simulink model "FMtest"  (R2025a)
settings: Solver=VariableStepAuto  StartTime=0.0  StopTime=3  RelTol=1e-3
undefined symbols (not defined in the file or in its folder): National_Instruments, PCIe
libraries: sldrtlib x5
settings Model: Creator=simmo536  LastModifiedBy=skaro014
settings DebuggingCC: UnconnectedInputMsg=warning  UnconnectedOutputMsg=warning  UnconnectedLineMsg=warning
settings ModelReferenceCC: EnableRefExpFcnMdlSchedulingChecks=on
settings RTWCC: GPUComputeCapability=3.5  DLArmComputeVersion=19.05

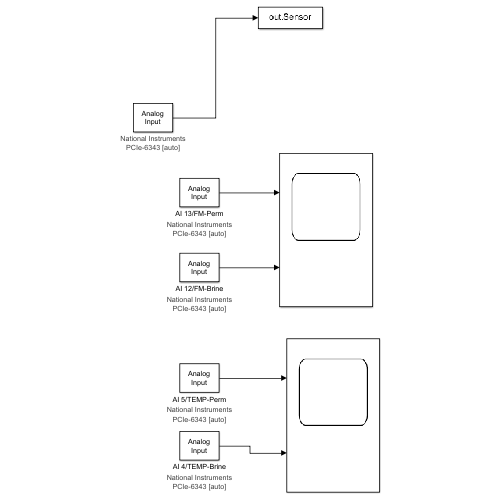
[thumbnail: Simulink's stored preview of the top-level diagram]
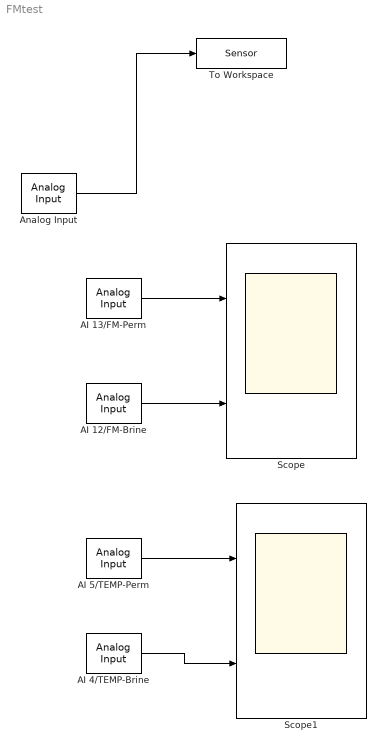
== system FMtest ==
  AI 12/FM-Brine : sldrtlib/Analog Input  SampleTime=0.01  MaxMissedTicks=inf  ShowMissedTicks=off  YieldWhenWaiting=off  DrvName=National_Instruments/PCIe-6343  DrvAddress=4294967295  DrvOptions=[0 0 0 0 0 0 0]  Channels=13  RangeMode=1  VoltRange=1  DataType=2
      settings: AttributesFormatString=National Instruments\nPCIe-6343 [auto]
  AI 13/FM-Perm : sldrtlib/Analog Input  SampleTime=0.01  MaxMissedTicks=inf  ShowMissedTicks=off  YieldWhenWaiting=off  DrvName=National_Instruments/PCIe-6343  DrvAddress=4294967295  DrvOptions=[0 0 0 0 0 0 0]  Channels=14  RangeMode=1  VoltRange=1  DataType=2
      settings: AttributesFormatString=National Instruments\nPCIe-6343 [auto]
  AI 4/TEMP-Brine : sldrtlib/Analog Input  SampleTime=0.01  MaxMissedTicks=inf  ShowMissedTicks=off  YieldWhenWaiting=on  DrvName=National_Instruments/PCIe-6343  DrvAddress=4294967295  DrvOptions=[0 0 0 0 0 0 0]  Channels=5  RangeMode=1  VoltRange=1  DataType=2
      settings: AttributesFormatString=National Instruments\nPCIe-6343 [auto]
  AI 5/TEMP-Perm : sldrtlib/Analog Input  SampleTime=0.01  MaxMissedTicks=inf  ShowMissedTicks=off  YieldWhenWaiting=on  DrvName=National_Instruments/PCIe-6343  DrvAddress=4294967295  DrvOptions=[0 0 0 0 0 0 0]  Channels=6  RangeMode=1  VoltRange=1  DataType=2
      settings: AttributesFormatString=National Instruments\nPCIe-6343 [auto]
  Analog Input : sldrtlib/Analog Input  SampleTime=0.1  MaxMissedTicks=inf  ShowMissedTicks=off  YieldWhenWaiting=on  DrvName=National_Instruments/PCIe-6343  DrvAddress=4294967295  DrvOptions=[0 4479 48128 3 3 3 3]  Channels=7  RangeMode=1  VoltRange=1  DataType=1
      settings: AttributesFormatString=National Instruments\nPCIe-6343 [auto]
  Scope : Scope  NumInputPorts=2
      settings: ActiveDisplayYMinimum=-9.46588  ActiveDisplayYMaximum=0.3586
  Scope1 : Scope  NumInputPorts=2
      settings: ActiveDisplayYMinimum=-4.84701  ActiveDisplayYMaximum=-1.62397
  To Workspace : ToWorkspace  VariableName=Sensor  SaveFormat=Timeseries  SampleTime=-1
  wires:
  AI 13/FM-Perm/1 -> Scope/1
  AI 12/FM-Brine/1 -> Scope/2
  AI 4/TEMP-Brine/1 -> Scope1/2
  AI 5/TEMP-Perm/1 -> Scope1/1
  Analog Input/1 -> To Workspace/1
